simulink model "svpwm"  (R2024b)
settings: Solver=VariableStepAuto  StartTime=0.0  StopTime=inf  RelTol=1e-3
libraries: simulink x2, spsDCVoltageSourceLib x1, spsPermanentMagnetSynchronousMachineLib x1, spsTwoLevelConverterLib x1, sps_lib x1
settings Model: Creator=alienware  LastModifiedBy=alienware

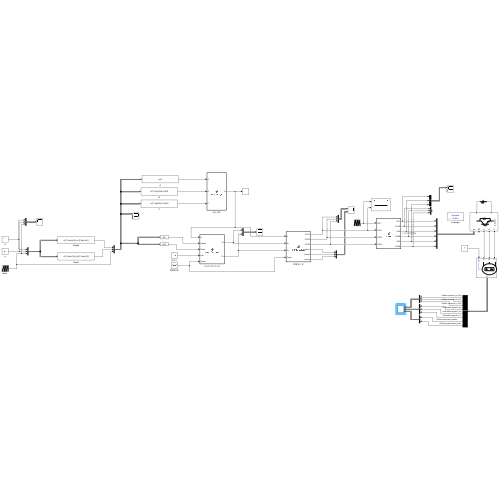
[thumbnail: Simulink's stored preview of the top-level diagram]
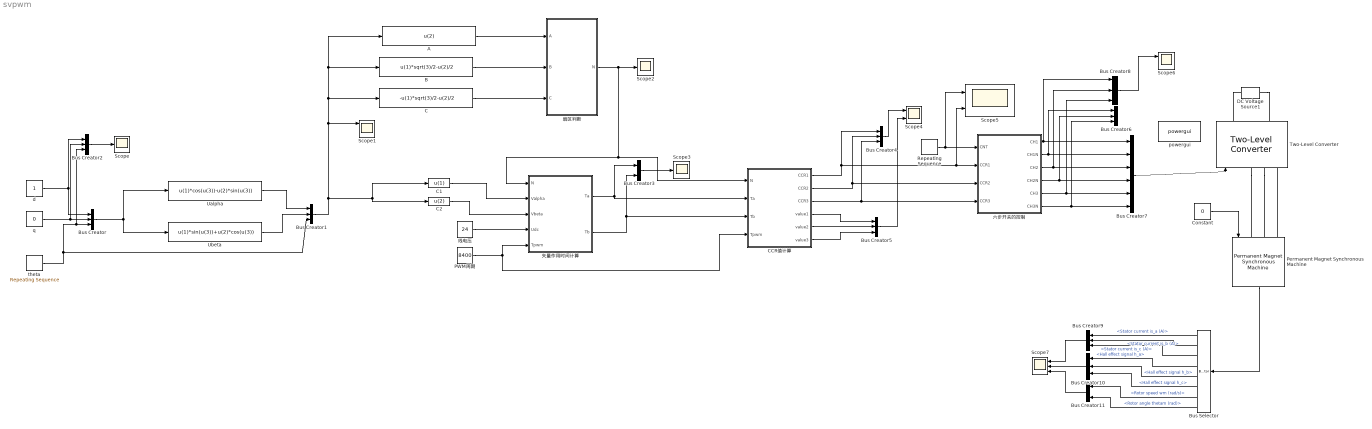
== system svpwm ==
  A : Fcn  Expr=u(2)
  B : Fcn  Expr=u(1)*sqrt(3)/2-u(2)/2
  Bus Creator{,1..2,4..6,8..10} (9 alike) : BusCreator  Inputs=3
  Bus Creator11 : BusCreator  Inputs=2
  Bus Creator3 : BusCreator  Inputs=2
  Bus Creator7 : BusCreator  Inputs=6
  Bus Selector : BusSelector  OutputSignals=Stator current is_a (A),Stator current is_b (A),Stator current is_c (A),Hall effect signal h_a,Hall effect signal h_b,Hall effect signal h_c,Rotor speed wm (rad/s),Rotor angle thetam (rad)
  C : Fcn  Expr=-u(1)*sqrt(3)/2-u(2)/2
  C1 : Fcn  Expr=u(1)
  C2 : Fcn  Expr=u(2)
  CCR值计算 : MATLAB Function  TreatAsAtomicUnit=on
  Constant : Constant  Value=0
  DC Voltage Source1 : spsDCVoltageSourceLib/DC Voltage Source  Amplitude=24  Measurements=None
  PWM周期 : Constant  Value=8400
  Permanent Magnet Synchronous Machine : spsPermanentMagnetSynchronousMachineLib/Permanent Magnet Synchronous Machine  NbPhases=3  FluxDistribution=Sinusoidal  RotorType=Round  MechanicalLoad=Torque Tm  PresetModel=No  ShowDetailedParameters=on  MeasurementBus=off  Resistance=0.0485  Inductance=8.5e-3  dqInductances=[8.5e-3,8.5e-3]  La=0.000395  MachineConstant=Flux linkage established by magnets (V.s)  Flux=0.1194  VoltageCst=86.6271  TorqueCst=0.7164  Flat=120  Mechanical=[0.0027 0.0004924 4 0]  PolePairs=4  InitialConditions=[0,0, 0,0]  InitialConditions5ph=[0 0 0 0 0 0]  RefAngle=Aligned with phase A axis (original Park)  IterativeDiscreteModel=Trapezoidal non iterative  TsBlock=-1  TsPowergui=0
  Repeating Sequence : simulink/Sources/Repeating Sequence  rep_seq_t=[0 0.00005 0.0001]  rep_seq_y=[0 4200 0]
  Scope : Scope
  Scope1 : Scope  NumInputPorts=3
  Scope2 : Scope
  Scope3 : Scope
  Scope4 : Scope  NumInputPorts=2
  Scope5 : Scope  NumInputPorts=2
  Scope6 : Scope  NumInputPorts=2
  Scope7 : Scope  NumInputPorts=3
  Two-Level Converter : spsTwoLevelConverterLib/Two-Level Converter  ModelType=Switching devices  Ron=1e-3  Rs=1e6  Cs=inf  Vforward=[0,0]  Ron_Diode=1e-3  Rs_Diode=1e6  Cs_Diode=inf  Vf_Diode=1e-3  Rs_CurrentSource=inf  Ron_ACsource=1e-3
      settings: LibrarySourceBlock=sps_lib/Power Electronics/Two-Level Converter
  Ualpha : Fcn  Expr=u(1)*cos(u(3))-u(2)*sin(u(3))
  Ubeta : Fcn  Expr=u(1)*sin(u(3))+u(2)*cos(u(3))
  d : Constant
  powergui : sps_lib/powergui  Priority=1  SimulationMode=Discrete  SampleTime=0.000001  frequency=60  Iterations=50  frequencyindice=0  Pbase=100e6  ErrMax=1e-4  UnitsV=kV  UnitsW=MW  buscounter=0  FunctionMessages=off  echomessages=off  EnableUseOfTLC=off  CurrentSourceSwitches=off  DisableSnubberDevices=off  DisableRonSwitches=off  DisableVfSwitches=off  DisplayEquations=off  AutomaticDiscreteSolvers=off  SolverType=Tustin/Backward Euler (TBE)  Interpol=off  ExternalGateDelay=off  methode=off  Ts=100  x0status=blocks  SPID=on  SwTol=0  HookPort=off  NonlinearTolerance=1e-4  nMaxIteration=100  ContinueOnMaxIteration=off  RestoreLinks=warning  ResistiveCurrentMeasurement=off  Frange=[0:2:500]  Ylog=off  Xlog=on  ShowGrid=off  save=off  variable=ZData  structure=0  ZoomFFT=off  StartTime=0.0  cycles=1  DisplayStyle=1  fundamental=60  FreqAxis=off  MaxFrequency=1000  frequencyindicesteady=1  RmsSteady=1  display=off
  q : Constant  Value=0
  "theta " : simulink/Sources/Repeating Sequence  rep_seq_t=[0 0.5]  rep_seq_y=[0 2*pi]
  六步开关的控制 : MATLAB Function  TreatAsAtomicUnit=on
  扇区判断 : MATLAB Function  TreatAsAtomicUnit=on
  矢量作用时间计算 : MATLAB Function  TreatAsAtomicUnit=on
  线电压 : Constant  Value=24
  wires:
  d/1 -> Bus Creator2/1, Bus Creator/1
  q/1 -> Bus Creator2/2, Bus Creator/2
  "theta "/1 -> Bus Creator2/3, Bus Creator/3, Bus Creator1/3
  Bus Creator/1 -> Ubeta/1, Ualpha/1
  Ualpha/1 -> Bus Creator1/1
  Ubeta/1 -> Bus Creator1/2
  Bus Creator2/1 -> Scope/1
  Bus Creator1/1 -> A/1, B/1, C/1, Scope1/1, C1/1, C2/1
  A/1 -> 扇区判断/1(A)
  B/1 -> 扇区判断/2(B)
  C/1 -> 扇区判断/3(C)
  扇区判断/1(N) -> Scope2/1, CCR值计算/1(N), 矢量作用时间计算/1(N)
  C1/1 -> 矢量作用时间计算/2(Valpha)
  C2/1 -> 矢量作用时间计算/3(Vbeta)
  线电压/1 -> 矢量作用时间计算/4(Udc)
  PWM周期/1 -> CCR值计算/4(Tpwm), 矢量作用时间计算/5(Tpwm)
  矢量作用时间计算/1(Ta) -> Bus Creator3/1, CCR值计算/2(Ta)
  矢量作用时间计算/2(Tb) -> Bus Creator3/2, CCR值计算/3(Tb)
  Bus Creator3/1 -> Scope3/1
  CCR值计算/3(CCR3) -> 六步开关的控制/4(CCR3), Bus Creator4/3
  CCR值计算/2(CCR2) -> Bus Creator4/2, 六步开关的控制/3(CCR2)
  CCR值计算/1(CCR1) -> Scope5/2, 六步开关的控制/2(CCR1), Bus Creator4/1
  Bus Creator4/1 -> Scope4/1
  CCR值计算/4(value1) -> Bus Creator5/1
  CCR值计算/5(value2) -> Bus Creator5/2
  CCR值计算/6(value3) -> Bus Creator5/3
  Bus Creator5/1 -> Scope4/2
  Repeating Sequence/1 -> 六步开关的控制/1(CNT), Scope5/1
  六步开关的控制/1(CH1) -> Bus Creator7/1, Bus Creator8/1
  六步开关的控制/2(CH1N) -> Bus Creator7/2, Bus Creator6/1
  六步开关的控制/3(CH2) -> Bus Creator7/3, Bus Creator8/2
  六步开关的控制/5(CH3) -> Bus Creator7/5, Bus Creator8/3
  六步开关的控制/4(CH2N) -> Bus Creator7/4, Bus Creator6/2
  六步开关的控制/6(CH3N) -> Bus Creator7/6, Bus Creator6/3
  Bus Creator8/1 -> Scope6/1
  Bus Creator7/1 -> Two-Level Converter/1
  Constant/1 -> Permanent Magnet Synchronous Machine/1
  Permanent Magnet Synchronous Machine/1 -> Bus Selector/1
  Bus Creator9/1 -> Scope7/1
  Bus Creator10/1 -> Scope7/2
  Bus Creator11/1 -> Scope7/3
  Bus Selector/1 -> Bus Creator9/1  "<Stator current is_a (A)>"
  Bus Selector/2 -> Bus Creator9/2  "<Stator current is_b (A)>"
  Bus Selector/3 -> Bus Creator9/3  "<Stator current is_c (A)>"
  Bus Selector/4 -> Bus Creator10/1  "<Hall effect signal h_a>"
  Bus Selector/5 -> Bus Creator10/2  "<Hall effect signal h_b>"
  Bus Selector/6 -> Bus Creator10/3  "<Hall effect signal h_c>"
  Bus Selector/7 -> Bus Creator11/1  "<Rotor speed wm (rad/s)>"
  Bus Selector/8 -> Bus Creator11/2  "<Rotor angle thetam (rad)>"
  connections:
  DC Voltage Source1/RConn1 -- Two-Level Converter/RConn1
  DC Voltage Source1/LConn1 -- Two-Level Converter/RConn2
  Permanent Magnet Synchronous Machine/LConn3 -- Two-Level Converter/LConn3
  Two-Level Converter/LConn2 -- Permanent Magnet Synchronous Machine/LConn2
  Two-Level Converter/LConn1 -- Permanent Magnet Synchronous Machine/LConn1

== matlab function svpwm/矢量作用时间计算 ==
  data: N input; Valpha input; Ta output; Vbeta input; Udc input; Tpwm input; Tb output
function [Ta,Tb] =VectorCalculate(N,Valpha,Vbeta,Udc,Tpwm )
Ta=double(0);
Tb=double(0);

X=(sqrt(3)*Tpwm)/Udc*Vbeta;
Y=(sqrt(3)*Tpwm)/Udc*((sqrt(3)/2)*Valpha-(1/2)*Vbeta);
Z=(sqrt(3)*Tpwm)/Udc*(-(sqrt(3)/2)*Valpha-(1/2)*Vbeta);

if N==3 %1%
    Ta=Y;
    Tb=X;

end
if N==1 %2%
    Ta=-Y;
    Tb=-Z;

end
if N==5 %3%
    Ta=X;
    Tb=Z;

end
if N==4 %4% 
    Ta=-X;
    Tb=-Y;

end
if N==6 %5%
    Ta=Z;
    Tb=Y;

end
if N==2 %6%
    Ta=-Z;
    Tb=-X;

end

== matlab function svpwm/扇区判断 ==
  data: A input; N output; B input; C input
function N =SectorJudge(A,B,C)


N=0;
if A>0
    N=N+1;
end
if B>0
    N=N+2; 
end
if C>0
    N=N+4;
end

== matlab function svpwm/CCR值计算 ==
  data: N input; Ta input; CCR1 output; Tb input; CCR2 output; CCR3 output; Tpwm input; value1 output; value2 output; value3 output
function [CCR1,CCR2,CCR3,value1,value2,value3] =CCRCalculate(N,Ta,Tb,Tpwm)
CCR1=double(0);
CCR2=double(0);
CCR3=double(0);
Ttemp=Ta+Tb;
if Ttemp>Tpwm
    Ta=Ta/Ttemp*Tpwm;
    Tb=Tb/Ttemp*Tpwm;
end
value1=(Tpwm-Ta-Tb)/4.0;
value2=value1+Ta/2.0;
value3=value2+Tb/2.0;
switch (N)
    case 3
        CCR1= value1;
        CCR2= value2;
        CCR3= value3;
     case 1
        CCR1= value2;
        CCR2= value1;
        CCR3= value3;
     case 5
        CCR1= value3 ;
        CCR2= value1;
        CCR3= value2;
     case 4
        CCR1= value3;
        CCR2= value2;
        CCR3= value1;
     case 6
        CCR1= value2;
        CCR2= value3;
        CCR3= value1;
     case 2
        CCR1= value1;
        CCR2= value3;
        CCR3= value2;
end

== matlab function svpwm/六步开关的控制 ==
  data: CNT input; CCR1 input; CH1 output; CH1N output; CCR2 input; CH2 output; CH2N output; CH3 output; CCR3 input; CH3N output
function [CH1,CH1N,CH2,CH2N,CH3,CH3N] =PWM(CNT,CCR1,CCR2,CCR3)
if CNT<CCR1
    CH1=0;
    CH1N=1;
else
    CH1=1;
    CH1N=0;
end
if CNT<CCR2
    CH2=0;
    CH2N=1;
else
    CH2=1;
    CH2N=0;
end
if CNT<CCR3
    CH3=0;
    CH3N=1;
else
    CH3=1;
    CH3N=0;
end
